simulink model "only_controller"  (R2023b)
settings: Solver=FixedStepAuto  StartTime=0.0  StopTime=10.0  FixedStep=Ts  RelTol=1e-3
values from neighbouring files (symbols this model uses):
  path = path * 0.1    [path_finder_waypoints.m]
undefined symbols (not defined in the file or in its folder): acceleration_limit, alpha, gear, Ki, Ki_turnrate, Kp, Kp_turnrate, taud, turn_acc_limit, wrad
libraries: robotalgslib x1
settings Model: Creator=simone  LastModifiedBy=simone
settings RTWCC: GenCodeOnly=on

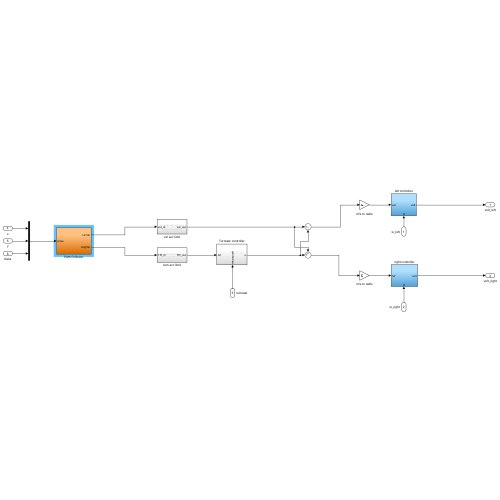
[thumbnail: Simulink's stored preview of the top-level diagram]
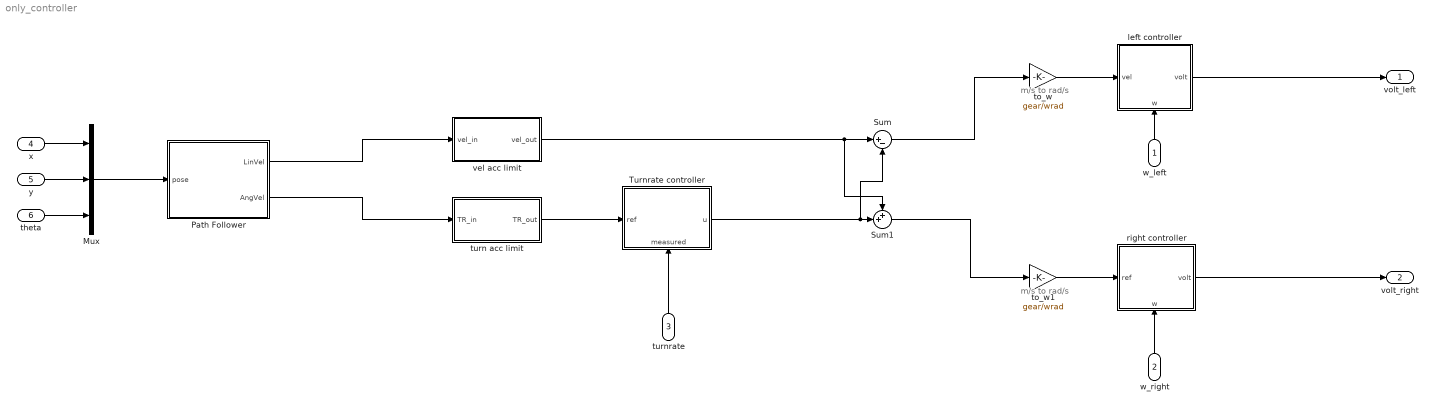
== system only_controller ==
  note: m/s to rad/s
  note: m/s to rad/s
  w_left : Inport
  w_right : Inport  Port=2
  turnrate : Inport  Port=3
  x : Inport  Port=4
  y : Inport  Port=5
  theta : Inport  Port=6
  Mux : Mux  Inputs=3
  Path Follower : Subsystem
  Sum : Sum  Inputs=|+-
  Sum1 : Sum  Inputs=++|
  Turnrate controller : Subsystem
      settings: PortSchema="{\"entries\":[{\"content\":{\"sides\":[{\"content\":{\"connectorIds\":[\"In1\"]},\"type\":\"ConnectorPlacement.EquallySpacedRectSide\",\"uuid\":\"3bde791d-a2ac-4d13-a51a-30874ee8f75a\"},{\"content\":{\"connectorIds\":[\"Out1\"],\"side\":\"RIGHT\"},\"type\":\"ConnectorPlacement.EquallySpacedRectSide\",\"uuid\":\"88ae4683-d3e7-483e-be55-3d26372f5fe2\"},{\"content\":{\"side\":\"TOP\"},\"type\":\"ConnectorPlacement.EquallySpacedRectSide\",\"uuid\":\"26752a72-f697-4de9-9dcd-1ca4cee0df39\"},{\"content\":{\"connectorIds\":[\"In2\"],\"side\":\"BOTTOM\"},\"type\":\"ConnectorPlacement.EquallySpacedRectSide\",\"uuid\":\"98a7b674-7c45-4a73-92a3-8750bdde1f36\"}]},\"type\":\"ConnectorPlacement.EquallySpacedConnector\",\"uuid\":\"d259c3e3-c5d7-42b6-881b-3a633aa969c6\"}],\"packageUris\":[\"http://schema.mathworks.com/mf0/Connector/R2020b\"],\"version\":\"1.0\"}"
  left controller : Subsystem
      settings: PortSchema="{\"entries\":[{\"content\":{\"sides\":[{\"content\":{\"connectorIds\":[\"In1\"]},\"type\":\"ConnectorPlacement.EquallySpacedRectSide\",\"uuid\":\"3bde791d-a2ac-4d13-a51a-30874ee8f75a\"},{\"content\":{\"connectorIds\":[\"Out1\"],\"side\":\"RIGHT\"},\"type\":\"ConnectorPlacement.EquallySpacedRectSide\",\"uuid\":\"88ae4683-d3e7-483e-be55-3d26372f5fe2\"},{\"content\":{\"side\":\"TOP\"},\"type\":\"ConnectorPlacement.EquallySpacedRectSide\",\"uuid\":\"26752a72-f697-4de9-9dcd-1ca4cee0df39\"},{\"content\":{\"connectorIds\":[\"In2\"],\"side\":\"BOTTOM\"},\"type\":\"ConnectorPlacement.EquallySpacedRectSide\",\"uuid\":\"8837b86a-35cd-4679-9975-e69b760c287c\"}]},\"type\":\"ConnectorPlacement.EquallySpacedConnector\",\"uuid\":\"d259c3e3-c5d7-42b6-881b-3a633aa969c6\"}],\"packageUris\":[\"http://schema.mathworks.com/mf0/Connector/R2020b\"],\"version\":\"1.0\"}"
  right controller : Subsystem
      settings: PortSchema="{\"entries\":[{\"content\":{\"sides\":[{\"content\":{\"connectorIds\":[\"In1\"]},\"type\":\"ConnectorPlacement.EquallySpacedRectSide\",\"uuid\":\"3bde791d-a2ac-4d13-a51a-30874ee8f75a\"},{\"content\":{\"connectorIds\":[\"Out1\"],\"side\":\"RIGHT\"},\"type\":\"ConnectorPlacement.EquallySpacedRectSide\",\"uuid\":\"88ae4683-d3e7-483e-be55-3d26372f5fe2\"},{\"content\":{\"side\":\"TOP\"},\"type\":\"ConnectorPlacement.EquallySpacedRectSide\",\"uuid\":\"26752a72-f697-4de9-9dcd-1ca4cee0df39\"},{\"content\":{\"connectorIds\":[\"In2\"],\"side\":\"BOTTOM\"},\"type\":\"ConnectorPlacement.EquallySpacedRectSide\",\"uuid\":\"1adabdfb-f360-4bb8-8b57-8160c74899b3\"}]},\"type\":\"ConnectorPlacement.EquallySpacedConnector\",\"uuid\":\"d259c3e3-c5d7-42b6-881b-3a633aa969c6\"}],\"packageUris\":[\"http://schema.mathworks.com/mf0/Connector/R2020b\"],\"version\":\"1.0\"}"
  to_w : Gain  Gain=gear/wrad
  to_w1 : Gain  Gain=gear/wrad
  turn acc limit : Subsystem
  vel acc limit : Subsystem
  volt_left : Outport
  volt_right : Outport  Port=2
  wires:
  Path Follower/2(AngVel) -> turn acc limit/1(TR_in)
  w_right/1 -> right controller/2(w)
  turnrate/1 -> Turnrate controller/2(measured)
  vel acc limit/1(vel_out) -> Sum1/1, Sum/1
  Turnrate controller/1(u) -> Sum/2, Sum1/2
  to_w1/1 -> right controller/1(ref)
  right controller/1(volt) -> volt_right/1
  left controller/1(volt) -> volt_left/1
  turn acc limit/1(TR_out) -> Turnrate controller/1(ref)
  Path Follower/1(LinVel) -> vel acc limit/1(vel_in)
  Sum1/1 -> to_w1/1
  w_left/1 -> left controller/2(w)
  to_w/1 -> left controller/1(vel)
  Sum/1 -> to_w/1
  x/1 -> Mux/1
  theta/1 -> Mux/3
  y/1 -> Mux/2
  Mux/1 -> Path Follower/1(pose)

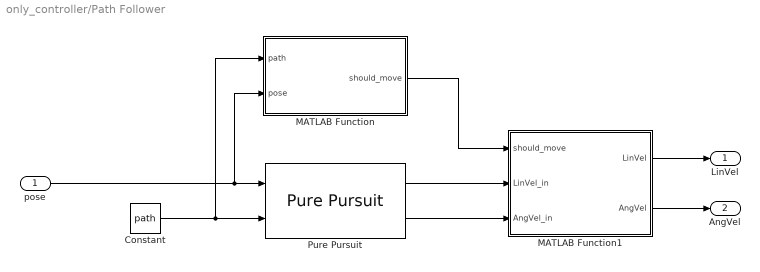
== system only_controller/Path Follower ==
  pose : Inport
  Constant : Constant  Value=path
  MATLAB Function : MATLAB Function  TreatAsAtomicUnit=on
  MATLAB Function1 : MATLAB Function  TreatAsAtomicUnit=on
  Pure Pursuit : robotalgslib/Pure Pursuit  DesiredLinearVelocity=vel_ref  MaxAngularVelocity=turn_acc_limit  LookaheadDistance=lookahead_dist  TargetDirPort=off  SimulateUsing=Code generation
      settings: LibrarySourceBlock=navlib/Control Algorithms/Pure Pursuit
  LinVel : Outport
  AngVel : Outport  Port=2
  wires:
  MATLAB Function/1(should_move) -> MATLAB Function1/1(should_move)
  pose/1 -> MATLAB Function/2(pose), Pure Pursuit/1
  MATLAB Function1/1(LinVel) -> LinVel/1
  MATLAB Function1/2(AngVel) -> AngVel/1
  Pure Pursuit/1 -> MATLAB Function1/2(LinVel_in)
  Pure Pursuit/2 -> MATLAB Function1/3(AngVel_in)
  Constant/1 -> MATLAB Function/1(path), Pure Pursuit/2

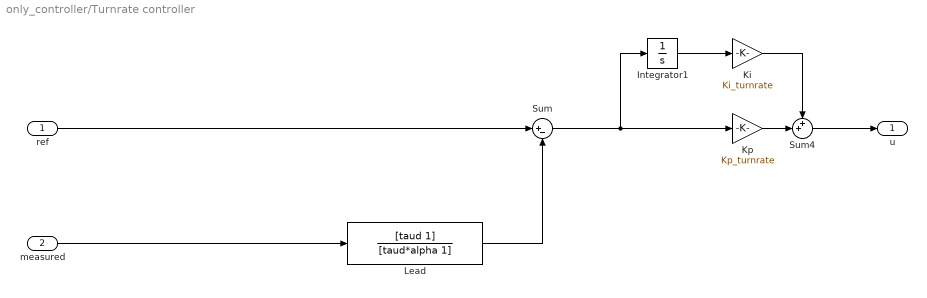
== system only_controller/Turnrate controller ==
  ref : Inport
  measured : Inport  Port=2
  Integrator1 : Integrator
  Ki : Gain  Gain=Ki_turnrate
  Kp : Gain  Gain=Kp_turnrate
  Lead : TransferFcn  Numerator=[taud 1]  Denominator=[taud*alpha 1]
  Sum : Sum  Inputs=|+-
  Sum4 : Sum  Inputs=++|
  u : Outport
  wires:
  ref/1 -> Sum/1
  Lead/1 -> Sum/2
  measured/1 -> Lead/1
  Sum4/1 -> u/1
  Sum/1 -> Integrator1/1, Kp/1
  Integrator1/1 -> Ki/1
  Ki/1 -> Sum4/1
  Kp/1 -> Sum4/2

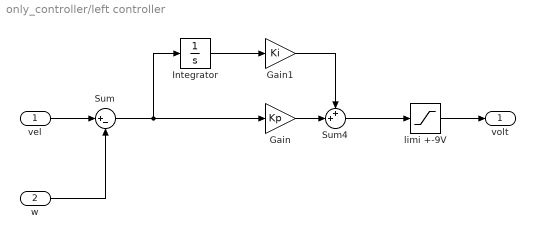
== system only_controller/left controller ==
  vel : Inport
  w : Inport  Port=2
  Gain : Gain  Gain=Kp
  Gain1 : Gain  Gain=Ki
  Integrator : Integrator
  Sum : Sum  Inputs=|+-
  Sum4 : Sum  Inputs=++|
  limi +-9V : Saturate  UpperLimit=9  LowerLimit=-9
  volt : Outport
  wires:
  Gain/1 -> Sum4/2
  Integrator/1 -> Gain1/1
  Gain1/1 -> Sum4/1
  vel/1 -> Sum/1
  w/1 -> Sum/2
  Sum/1 -> Integrator/1, Gain/1
  Sum4/1 -> limi +-9V/1
  limi +-9V/1 -> volt/1

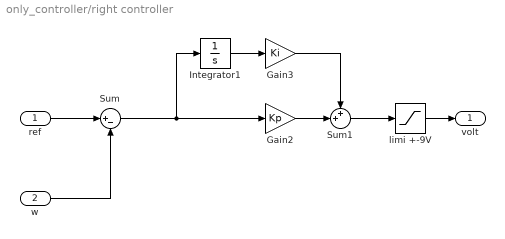
== system only_controller/right controller ==
  ref : Inport
  w : Inport  Port=2
  Gain2 : Gain  Gain=Kp
  Gain3 : Gain  Gain=Ki
  Integrator1 : Integrator
  Sum : Sum  Inputs=|+-
  Sum1 : Sum  Inputs=++|
  limi +-9V : Saturate  UpperLimit=9  LowerLimit=-9
  volt : Outport
  wires:
  Integrator1/1 -> Gain3/1
  Gain2/1 -> Sum1/2
  Gain3/1 -> Sum1/1
  Sum/1 -> Integrator1/1, Gain2/1
  ref/1 -> Sum/1
  w/1 -> Sum/2
  Sum1/1 -> limi +-9V/1
  limi +-9V/1 -> volt/1

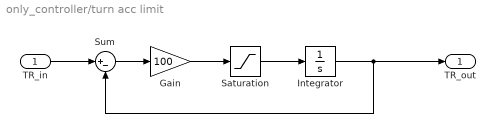
== system only_controller/turn acc limit ==
  TR_in : Inport
  Gain : Gain  Gain=100
  Integrator : Integrator
  Saturation : Saturate  UpperLimit=turn_acc_limit  LowerLimit=-turn_acc_limit
  Sum : Sum  Inputs=|+-
  TR_out : Outport
  wires:
  TR_in/1 -> Sum/1
  Sum/1 -> Gain/1
  Gain/1 -> Saturation/1
  Saturation/1 -> Integrator/1
  Integrator/1 -> Sum/2, TR_out/1

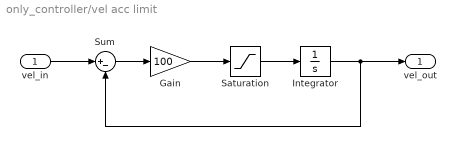
== system only_controller/vel acc limit ==
  vel_in : Inport
  Gain : Gain  Gain=100
  Integrator : Integrator
  Saturation : Saturate  UpperLimit=acceleration_limit  LowerLimit=-acceleration_limit
  Sum : Sum  Inputs=|+-
  vel_out : Outport
  wires:
  vel_in/1 -> Sum/1
  Sum/1 -> Gain/1
  Gain/1 -> Saturation/1
  Saturation/1 -> Integrator/1
  Integrator/1 -> Sum/2, vel_out/1

== matlab function only_controller/Path Follower/MATLAB Function1 ==
  data: should_move input; LinVel output; LinVel_in input; AngVel_in input; AngVel output
function [LinVel, AngVel] = get_res(should_move, LinVel_in, AngVel_in)

if should_move
    LinVel = LinVel_in;
    AngVel = AngVel_in;
else
    LinVel = 0;
    AngVel = 0;
end

== matlab function only_controller/Path Follower/MATLAB Function ==
  data: path input; should_move output; pose input
function should_move = are_we_at_goal(path, pose)

pose = pose([1 2], :)';
robotGoal = path(end, :);

goalRadius = 0.05;
distanceToGoal = norm(pose - robotGoal);

if distanceToGoal < goalRadius
    should_move = 0;
else
    should_move = 1;
end
